simulink model "delay_core_test"  (Simulink 7.0)
settings: Solver=ode45  StartTime=0.0  StopTime=100+2^15  RelTol=1e-3
libraries: xbsIndex_r4 x25, simulink x5, beamform x2
settings Model: Creator=mdexter  LastModifiedBy=mdexter

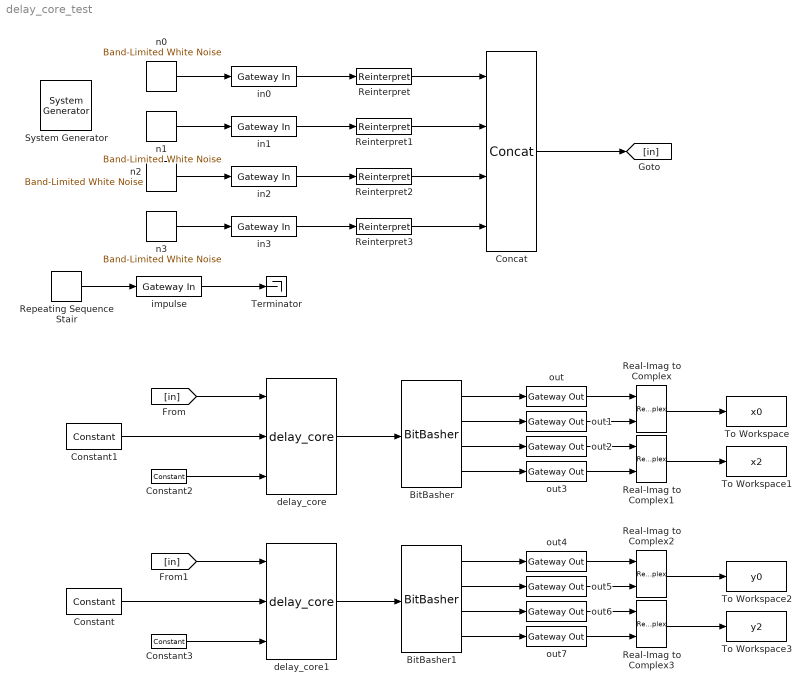
== system delay_core_test ==
  " System Generator" : xbsIndex_r4/ System Generator  Tag=genX  SystemSampleTime=-1  xilinxfamily=virtex2p  part=xc2vp50  speed=-7  package=ff1152  synthesis_tool=XST  clock_wrapper=Clock Enables  directory=./delay_core  testbench=off  simulink_period=1  sysclk_period=100  dcm_input_clock_period=100  incr_netlist=off  trim_vbits=Everywhere in SubSystem  dbl_ovrd=According to Block Masks  core_generation=According to Block Masks  run_coregen=off  deprecated_control=off  eval_field=0  block_type=sysgen
      settings: block_version=10.1.3
  BitBasher : xbsIndex_r4/BitBasher  bitexpr=|  display_expr=off  sr_1=1  arith_type1="Signed  (2's comp)"  bin_pt1=0  sr_2=2  arith_type2="Signed  (2's comp)"  bin_pt2=0  sr_3=3  arith_type3="Signed  (2's comp)"  bin_pt3=0  sr_4=4  arith_type4="Signed  (2's comp)"  bin_pt4=0  dbl_ovrd=off  block_type=bitbasher
      | <html><head><meta name="qrichtext" content="1" /><style type="text/css">
      | p, li { white-space: pre-wrap; }
      | </style></head><body style=" font-family:'MS Shell Dlg 2'; font-size:8.25pt; font-weight:400; font-style:normal;">
      | <p style=" margin-top:12px; margin-bottom:12px; margin-left:0px; margin-right:0px; -qt-block-indent:0; text-indent:0px; font-family:'MS Shell Dlg'; font-size:8pt;">z0_re={in[31:24]}<br />z0_im={in[23:16]}<br />z2_re={in[15:8]}<br />z2_im={in[7:0]}<br /></p></body></html>
      settings: block_version=10.1.3
  BitBasher1 : xbsIndex_r4/BitBasher  bitexpr=|  display_expr=off  sr_1=1  arith_type1="Signed  (2's comp)"  bin_pt1=0  sr_2=2  arith_type2="Signed  (2's comp)"  bin_pt2=0  sr_3=3  arith_type3="Signed  (2's comp)"  bin_pt3=0  sr_4=4  arith_type4="Signed  (2's comp)"  bin_pt4=0  dbl_ovrd=off  block_type=bitbasher
      | <html><head><meta name="qrichtext" content="1" /><style type="text/css">
      | p, li { white-space: pre-wrap; }
      | </style></head><body style=" font-family:'MS Shell Dlg 2'; font-size:8.25pt; font-weight:400; font-style:normal;">
      | <p style=" margin-top:12px; margin-bottom:12px; margin-left:0px; margin-right:0px; -qt-block-indent:0; text-indent:0px; font-family:'MS Shell Dlg'; font-size:8pt;">z0_re={in[31:24]}<br />z0_im={in[23:16]}<br />z2_re={in[15:8]}<br />z2_im={in[7:0]}<br /></p></body></html>
      settings: block_version=10.1.3
  Concat : xbsIndex_r4/Concat  num_inputs=4  dbl_ovrd=off  block_type=concat
      settings: block_version=10.1.3
  Constant : xbsIndex_r4/Constant  arith_type=Unsigned  const=1+15/16  n_bits=17  bin_pt=4  explicit_period=on  period=1  equ=P=C  opselect=C  inp2=PCIN>>17  opr=+  inp1=P  carry=CIN  dbl_ovrd=off  block_type=constant
  Constant1 : xbsIndex_r4/Constant  arith_type=Unsigned  const=0  n_bits=17  bin_pt=4  explicit_period=on  period=1  equ=P=C  opselect=C  inp2=PCIN>>17  opr=+  inp1=P  carry=CIN  dbl_ovrd=off  block_type=constant
  Constant2 : xbsIndex_r4/Constant  arith_type=Boolean  const=0  n_bits=17  bin_pt=4  explicit_period=on  period=1  equ=P=C  opselect=C  inp2=PCIN>>17  opr=+  inp1=P  carry=CIN  dbl_ovrd=off  block_type=constant
  Constant3 : xbsIndex_r4/Constant  arith_type=Boolean  const=0  n_bits=17  bin_pt=4  explicit_period=on  period=1  equ=P=C  opselect=C  inp2=PCIN>>17  opr=+  inp1=P  carry=CIN  dbl_ovrd=off  block_type=constant
  Real-Imag to Complex{,1..3} (4 alike) : RealImagToComplex
  Reinterpret{,1..3} (4 alike) : xbsIndex_r4/Reinterpret  force_arith_type=on  arith_type=Unsigned  force_bin_pt=on  bin_pt=0  block_type=reinterpret
      settings: infoedit="Changes signal type without altering the binary representation.   You can changed the signal between signed and unsigned, and relocate the binary point.<P><P>Hardware notes: In hardware this block costs nothing.<P><P>Example:  Suppose the input is 6 bits wide, signed, with 2 fractional bits, and the output is forced to unsigned with 0 fractional bits.  Then an input of -2.0 (1110.00 in binary 2's complement) becomes an output of 56 (111000 in binary)."  block_version=10.1.3
  Repeating Sequence Stair : simulink/Sources/Repeating Sequence Stair  SystemSampleTime=-1  OutValues=[0 1 zeros(1,1e4)]*2^31  tsamp=1  OutMin=[]  OutMax=[]  OutDataTypeStr=float('double')  OutputDataTypeScalingMode=Specify via dialog  OutDataType=float('double')  ConRadixGroup=Best Precision: Vector-wise  OutScaling=2^-12
  Terminator : Terminator
  To Workspace : ToWorkspace  VariableName=x0  SampleTime=-1  SaveFormat=Array
  To Workspace1 : ToWorkspace  VariableName=x2  SampleTime=-1  SaveFormat=Array
  To Workspace2 : ToWorkspace  VariableName=y0  SampleTime=-1  SaveFormat=Array
  To Workspace3 : ToWorkspace  VariableName=y2  SampleTime=-1  SaveFormat=Array
  delay_core : beamform/delay_core  SystemSampleTime=-1
  delay_core1 : beamform/delay_core  SystemSampleTime=-1
  impulse : xbsIndex_r4/Gateway In  arith_type=Unsigned  n_bits=32  bin_pt=0  quantization="Round  (unbiased: +/- Inf)"  overflow=Saturate  period=1  dbl_ovrd=off  timing_constraint=None  locs_specified=off  LOCs={}  block_type=gatewayin
      settings: infoedit="Gateway in block.  Converts inputs of type Simulink integer, double and fixed point to  Xilinx fixed point type.<P><P>Hardware notes:  In hardware these blocks become top level input ports."  block_version=10.1.3
  in{0..3} (4 alike) : xbsIndex_r4/Gateway In  arith_type="Signed  (2's comp)"  n_bits=8  bin_pt=0  quantization="Round  (unbiased: +/- Inf)"  overflow=Saturate  period=1  dbl_ovrd=off  timing_constraint=None  locs_specified=off  LOCs={}  block_type=gatewayin
      settings: infoedit="Gateway in block.  Converts inputs of type Simulink integer, double and fixed point to  Xilinx fixed point type.<P><P>Hardware notes:  In hardware these blocks become top level input ports."  block_version=10.1.3
  n0 : simulink/Sources/Band-Limited White Noise  SystemSampleTime=-1  Cov=13^2  Ts=1  seed=[23341]
  n1 : simulink/Sources/Band-Limited White Noise  SystemSampleTime=-1  Cov=13^2  Ts=1  seed=[11111]
  n2 : simulink/Sources/Band-Limited White Noise  SystemSampleTime=-1  Cov=13^2  Ts=1  seed=[22222]
  n3 : simulink/Sources/Band-Limited White Noise  SystemSampleTime=-1  Cov=13^2  Ts=1  seed=[33333]
  out{,1..7} (8 alike) : xbsIndex_r4/Gateway Out  hdl_port=off  timing_constraint=None  locs_specified=off  LOCs={}  block_type=gatewayout
      settings: infoedit="Gateway out block.  Converts Xilinx fixed point inputs into ouputs of type Simulink integer, double, or fixed point.<P><P>Hardware notes:  In hardware these blocks become top level output ports or are discarded, depending on how they are configured."  block_version=10.1.3
  wires:
  [in] -> delay_core/1
  delay_core/1 -> BitBasher/1
  Constant1/1 -> delay_core/2
  Constant2/1 -> delay_core/3
  in0/1 -> Reinterpret/1
  in1/1 -> Reinterpret1/1
  in2/1 -> Reinterpret2/1
  in3/1 -> Reinterpret3/1
  n0/1 -> in0/1
  n1/1 -> in1/1
  n2/1 -> in2/1
  n3/1 -> in3/1
  Reinterpret/1 -> Concat/1
  Reinterpret1/1 -> Concat/2
  Reinterpret2/1 -> Concat/3
  Reinterpret3/1 -> Concat/4
  Constant/1 -> delay_core1/2
  [in] -> delay_core1/1
  Constant3/1 -> delay_core1/3
  BitBasher/1 -> out/1
  BitBasher/2 -> out1/1
  BitBasher/3 -> out2/1
  BitBasher/4 -> out3/1
  out/1 -> Real-Imag to Complex/1
  out1/1 -> Real-Imag to Complex/2
  out2/1 -> Real-Imag to Complex1/1
  out3/1 -> Real-Imag to Complex1/2
  Real-Imag to Complex/1 -> To Workspace/1
  Real-Imag to Complex1/1 -> To Workspace1/1
  delay_core1/1 -> BitBasher1/1
  BitBasher1/1 -> out4/1
  BitBasher1/2 -> out5/1
  BitBasher1/3 -> out6/1
  BitBasher1/4 -> out7/1
  out4/1 -> Real-Imag to Complex2/1
  out5/1 -> Real-Imag to Complex2/2
  out6/1 -> Real-Imag to Complex3/1
  out7/1 -> Real-Imag to Complex3/2
  Real-Imag to Complex2/1 -> To Workspace2/1
  Real-Imag to Complex3/1 -> To Workspace3/1
  Concat/1 -> [in]
  Repeating Sequence Stair/1 -> impulse/1
  impulse/1 -> Terminator/1
